simulink model "q2_PAM_simulink_model"  (R2020b)
settings: Solver=VariableStepAuto  StartTime=0.0  StopTime=10.0  RelTol=1e-3
values from neighbouring files (symbols this model uses):
  Tb = Ts/K    [q2_a.m]    (also in q2_b.m)
libraries: commutil2 x2, commdigbbndam3 x2, commchan3 x1, commrandsrc3 x1, commsink2 x1
settings Model: Creator=aykut  LastModifiedBy=aykut

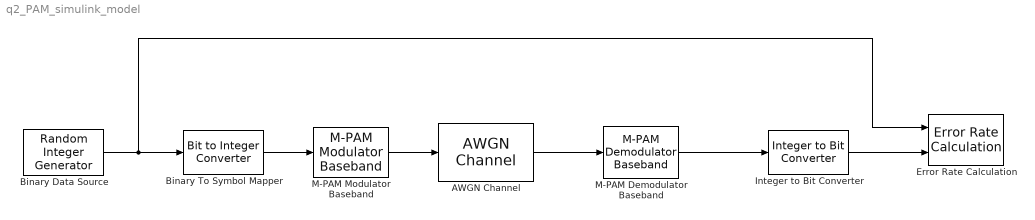
== system q2_PAM_simulink_model ==
  AWGN Channel : commchan3/AWGN Channel  InputProcessing=Columns as channels (frame based)  seed=67  noiseMode="Signal to noise ratio  (Eb/No)"  EbNodB=EbNOdB  EsNodB=10  SNRdB=10  bitsPerSym=K  Ps=1  Tsym=Ts  variance=1
  Binary Data Source : commrandsrc3/Random Integer Generator  SetSize=2  SeedSource=Auto  Seed=0  SampleTime=Tb  SamplesPerFrame=Nbps  OutputDataType=double  SimulateUsing=Interpreted execution
  Binary To Symbol Mapper : commutil2/Bit to Integer Converter  nbits=K  bitOrder=MSB first  signedOutputValues=Unsigned  outDtype=Inherit via internal rule  outDtypeSigned=Inherit via internal rule
  Error Rate Calculation : commsink2/Error Rate Calculation  N=0  st_delay=0  cp_mode=Entire frame  subframe=[]  PMode=Workspace  WsName=ChannelError  RsMode2=off  stop=off  numErr=100  maxBits=1e6
  Integer to Bit Converter : commutil2/Integer to Bit Converter  nbits=K  signedInputValues=Unsigned  bitOrder=MSB first  outDtype=Inherit via internal rule
  M-PAM Demodulator Baseband : commdigbbndam3/M-PAM Demodulator Baseband  M=M  OutType=Integer  Dec=Gray  PowType=Average Power  MinDist=2  AvgPow=1  PeakPow=1  outDtype1=Inherit via internal rule  outDtype2=Inherit via internal rule  denormFactorWordLen=16  denormFactorDataTypeStr=Inherit: Same word length as input  denormFactorLastDataTypeStr=Inherit: Same word length as input  prodOutWordLen=16  prodOutRoundingMode=Floor  prodOutOverflowMode=Wrap  prodOutOvFlMode=off  prodOutOvFlModeLastStrValue=off  sumWordLen=16
      settings: SourceProductBaseCode=CM
  M-PAM Modulator Baseband : commdigbbndam3/M-PAM Modulator Baseband  M=M  InType=Integer  Enc=Gray  PowType=Average Power  MinDist=2  AvgPow=1  PeakPow=1  outDtype=double  outWordLen=16  outUDDataType=sfix(16)  outFracLenMode=Best precision  outFracLen=15  outDataTypeStr=double  outLastDataTypeStr=double
      settings: SourceProductBaseCode=CM
  wires:
  M-PAM Modulator Baseband/1 -> AWGN Channel/1
  Integer to Bit Converter/1 -> Error Rate Calculation/2
  Binary Data Source/1 -> Error Rate Calculation/1, Binary To Symbol Mapper/1
  M-PAM Demodulator Baseband/1 -> Integer to Bit Converter/1
  AWGN Channel/1 -> M-PAM Demodulator Baseband/1
  Binary To Symbol Mapper/1 -> M-PAM Modulator Baseband/1
